simulink model "ModeleSimulinkQ20_2016a"  (R2016a)
settings: Solver=VariableStepAuto  SolverMode=SingleTasking  StartTime=0.0  StopTime=500  RelTol=1e-3
values from neighbouring files (symbols this model uses):
  qdf = [0 1 0 0 0 0]'    [TP2.m]
  qdi = [-1 0 -1 -1 -1 -1]'    [TP2.m]
libraries: simulink x1
settings Model: Creator=davide  LastModifiedBy=davide
settings DataIOCC: ReturnWorkspaceOutputs=on
settings DebuggingCC: SFUnexpectedBacktrackingDiag=error  SFNoUnconditionalDefaultTransitionDiag=error
settings SFSimCC: SimUseLocalCustomCode=on
settings RTWCC: RTWUseLocalCustomCode=on
settings GRTTargetCC: TargetLangStandard=C99 (ISO)  GeneratePreprocessorConditionals=Use local settings
settings ConfigComp: CovMetricSettings=dwe  CovHtmlReporting=off  CovSaveCumulativeToWorkspaceVar=off  CovSaveSingleToWorkspaceVar=off  CovExternalEMLEnable=on

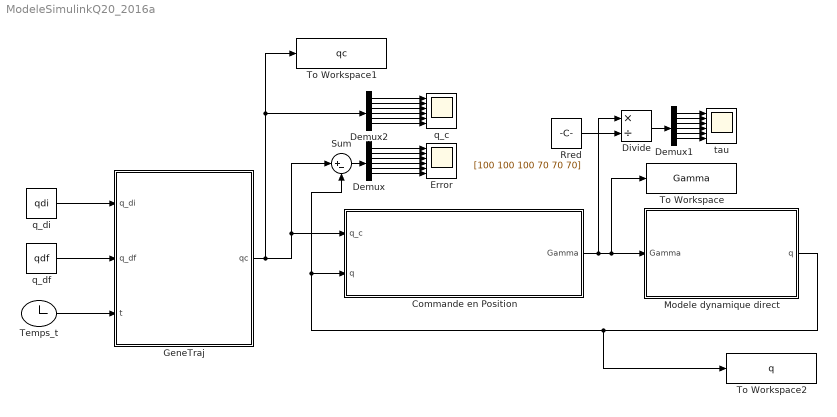
== system ModeleSimulinkQ20_2016a ==
  Commande en Position : Subsystem
  Demux : Demux  Outputs=6
  Demux1 : Demux  Outputs=6
  Demux2 : Demux  Outputs=6
  Divide : Product  Inputs=*/
  Error : Scope  NumInputPorts=6
  GeneTraj : MATLAB Function  TreatAsAtomicUnit=on
  Modele dynamique direct : Subsystem
  Rred : Constant  Value=[100 100 100 70 70 70]
  Sum : Sum  Inputs=|+-
  "Temps_t " : Clock
  To Workspace : ToWorkspace  VariableName=Gamma  SaveFormat=Timeseries  SampleTime=-1
  To Workspace1 : ToWorkspace  VariableName=qc  SaveFormat=Timeseries  SampleTime=-1
  To Workspace2 : ToWorkspace  VariableName=q  SaveFormat=Timeseries  SampleTime=-1
  q_c : Scope  NumInputPorts=6
  "q_df " : Constant  Value=qdf  VectorParams1D=off
  q_di : Constant  Value=qdi  VectorParams1D=off
  tau : Scope  NumInputPorts=6
  wires:
  GeneTraj/1(qc) -> Demux2/1, To Workspace1/1, Sum/1, Commande en Position/1(q_c)
  "Temps_t "/1 -> GeneTraj/3(t)
  "q_df "/1 -> GeneTraj/2(q_df)
  q_di/1 -> GeneTraj/1(q_di)
  Commande en Position/1(Gamma) -> Divide/1, To Workspace/1, Modele dynamique direct/1(Gamma)
  Modele dynamique direct/1(q) -> To Workspace2/1, Sum/2, Commande en Position/2(q)
  Sum/1 -> Demux/1
  Demux/4 -> Error/4
  Demux/1 -> Error/1
  Demux/2 -> Error/2
  Demux/3 -> Error/3
  Demux/5 -> Error/5
  Demux/6 -> Error/6
  Demux2/2 -> q_c/2
  Demux2/6 -> q_c/6
  Demux2/4 -> q_c/4
  Demux2/5 -> q_c/5
  Demux2/3 -> q_c/3
  Demux2/1 -> q_c/1
  Demux1/3 -> tau/3
  Demux1/5 -> tau/5
  Demux1/4 -> tau/4
  Demux1/2 -> tau/2
  Demux1/6 -> tau/6
  Demux1/1 -> tau/1
  Divide/1 -> Demux1/1
  Rred/1 -> Divide/2

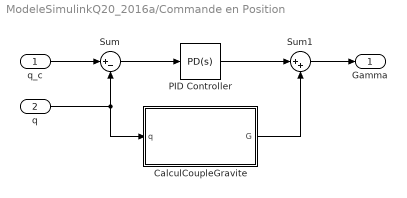
== system ModeleSimulinkQ20_2016a/Commande en Position ==
  q_c : Inport
  q : Inport  Port=2
  CalculCoupleGravite : MATLAB Function  TreatAsAtomicUnit=on
  PID Controller : simulink/Continuous/PID Controller  Controller=PD  Form=Parallel  TimeDomain=Continuous-time  SampleTime=-1  IntegratorMethod=Forward Euler  FilterMethod=Forward Euler  ControllerParametersSource=internal  P=1  I=0  D=0.4  UseFilter=on  N=100  InitialConditionSource=internal  InitialConditionForIntegrator=0  InitialConditionForFilter=0  DifferentiatorICPrevScaledInput=0  ExternalReset=none  TrackingMode=off  Kt=1  LimitOutput=off  UpperSaturationLimit=inf  LowerSaturationLimit=-inf  LinearizeAsGain=on  AntiWindupMode=none  Kb=1  POutMin=[]  POutMax=[]  IOutMin=[]  IOutMax=[]  DOutMin=[]  DOutMax=[]  NOutMin=[]  NOutMax=[]  SumOutMin=[]  SumOutMax=[]  SaturationOutMin=[]  SaturationOutMax=[]  PParamMin=[]  PParamMax=[]  IParamMin=[]  IParamMax=[]  DParamMin=[]  DParamMax=[]  NParamMin=[]  NParamMax=[]  KbParamMin=[]  KbParamMax=[]  KtParamMin=[]  KtParamMax=[]  KbOutMin=[]  KbOutMax=[]  KtOutMin=[]  KtOutMax=[]  IntegratorOutMin=[]  IntegratorOutMax=[]  FilterOutMin=[]  FilterOutMax=[]  SumI1OutMin=[]  SumI1OutMax=[]  SumI2OutMin=[]  SumI2OutMax=[]  SumI3OutMin=[]  SumI3OutMax=[]  SumDOutMin=[]  SumDOutMax=[]  DifferentiatorOutMin=[]  DifferentiatorOutMax=[]  IntegratorContinuousStateAttributes=''  IntegratorStateMustResolveToSignalObject=off  IntegratorRTWStateStorageClass=Auto  FilterContinuousStateAttributes=''  FilterStateMustResolveToSignalObject=off  FilterRTWStateStorageClass=Auto
  Sum : Sum  Inputs=|+-
  Sum1 : Sum  Inputs=|++
  Gamma : Outport
  wires:
  q/1 -> CalculCoupleGravite/1(q), Sum/2
  q_c/1 -> Sum/1
  Sum/1 -> PID Controller/1
  PID Controller/1 -> Sum1/1
  Sum1/1 -> Gamma/1
  CalculCoupleGravite/1(G) -> Sum1/2

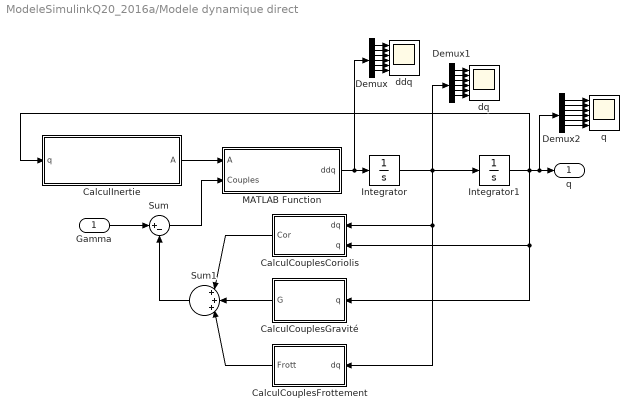
== system ModeleSimulinkQ20_2016a/Modele dynamique direct ==
  Gamma : Inport
  CalculCouplesCoriolis : MATLAB Function  TreatAsAtomicUnit=on
  CalculCouplesFrottement : MATLAB Function  TreatAsAtomicUnit=on
  CalculCouplesGravité : MATLAB Function  TreatAsAtomicUnit=on
  CalculInertie : MATLAB Function  TreatAsAtomicUnit=on
  Demux : Demux  Outputs=6
  Demux1 : Demux  Outputs=6
  Demux2 : Demux  Outputs=6
  Integrator : Integrator
  Integrator1 : Integrator  InitialCondition=[-1 0 -1 -1 -1 -1]'
  MATLAB Function : MATLAB Function  TreatAsAtomicUnit=on
  Sum : Sum  Inputs=|+-
  Sum1 : Sum  Inputs=|+++|
  "ddq " : Scope  NumInputPorts=6
  dq : Scope  NumInputPorts=6
  "q " : Scope  NumInputPorts=6
  q : Outport
  wires:
  Integrator1/1 -> CalculCouplesGravité/1(q), CalculCouplesCoriolis/2(q), CalculInertie/1(q), Demux2/1, q/1
  Integrator/1 -> CalculCouplesFrottement/1(dq), CalculCouplesCoriolis/1(dq), Demux1/1, Integrator1/1
  Gamma/1 -> Sum/1
  CalculInertie/1(A) -> MATLAB Function/1(A)
  Sum/1 -> MATLAB Function/2(Couples)
  MATLAB Function/1(ddq) -> Demux/1, Integrator/1
  Demux/1 -> "ddq "/1
  Demux/2 -> "ddq "/2
  Demux/3 -> "ddq "/3
  Demux/4 -> "ddq "/4
  Demux/5 -> "ddq "/5
  Demux/6 -> "ddq "/6
  Demux1/2 -> dq/2
  Demux1/4 -> dq/4
  Demux1/6 -> dq/6
  Demux1/3 -> dq/3
  Demux1/5 -> dq/5
  Demux1/1 -> dq/1
  Demux2/4 -> "q "/4
  Demux2/1 -> "q "/1
  Demux2/6 -> "q "/6
  Demux2/5 -> "q "/5
  Demux2/2 -> "q "/2
  Demux2/3 -> "q "/3
  Sum1/1 -> Sum/2
  CalculCouplesFrottement/1(Frott) -> Sum1/3
  CalculCouplesGravité/1(G) -> Sum1/2
  CalculCouplesCoriolis/1(Cor) -> Sum1/1

== matlab function ModeleSimulinkQ20_2016a/Commande en Position/CalculCoupleGravite ==
  data: q input; G output
function G = CalculCoupleGravite(q)

    %Parametres
    m=[15 10 1 7 1 0.5];
    x_G1 = 0; y_G1 = 0; z_G1 = -0.25;
    x_G2 = 0.35; y_G2 = 0; z_G2 = 0;
    x_G3 = 0; y_G3 = -0.1; z_G3 = 0;
    x_G4 = 0; y_G4 = 0; z_G4 = 0;
    x_G5 = 0; y_G5 = 0; z_G5 = 0;
    x_G6 = 0; y_G6 = 0; z_G6 = 0;
    x_G = [x_G1 x_G2 x_G3 x_G4 x_G5 x_G6];
    y_G = [y_G1 y_G2 y_G3 y_G4 y_G5 y_G6];
    z_G = [z_G1 z_G2 z_G3 z_G4 z_G5 z_G6];

    d = [0 0 0.7 0 0 0];
    r = [0.5 0 0 0.2 0 0];
    alpha = [0 pi/2 0 pi/2 -pi/2 pi/2];
    theta = [q(1) q(2) q(3)+pi/2 q(4) q(5) q(6)];

    % Calcul des matrices jacobiennes de chacun des corps
    [OJv_Gi, ~] = CalculMatriceJacobienneGi(alpha, d, theta, r, x_G, y_G, z_G);

    %Vecteur gravité exprimé dans R0
    g = [0 0 -9.81]';

    %Calcul du couple de gravité produit par les corps
    G = zeros(length(theta), 1);
    
    for i = 1:length(m)
        G = G - OJv_Gi(:,:,i)'*m(i)*g;
    end
end

== matlab function ModeleSimulinkQ20_2016a/GeneTraj ==
  data: q_di input; qc output; q_df input; t input
function qc = GeneTraj(q_di, q_df, t)
    
    tf = 500;
     
    D = (q_df - q_di);
    
    r = 10 * (t/tf)^3 - 15 * (t/tf)^4 + 6 * (t/tf)^5;
    
    qc = q_di + r*D;
end

== matlab function ModeleSimulinkQ20_2016a/Modele dynamique direct/CalculCouplesCoriolis ==
  data: dq input; q input; Cor output
function Cor = fcn(dq, q)

    Cor = CalculCoupleCoriolisCentrifuge(q, dq)'; 

end

== matlab function ModeleSimulinkQ20_2016a/Modele dynamique direct/CalculInertie ==
  data: q input; A output
function A = CalculMatriceInertie(q)


    %Parametres
    m=[15 10 1 7 1 0.5];
    
    x_G1 = 0; y_G1 = 0; z_G1 = -0.25;
    x_G2 = 0.35; y_G2 = 0; z_G2 = 0;
    x_G3 = 0; y_G3 = -0.1; z_G3 = 0;
    x_G4 = 0; y_G4 = 0; z_G4 = 0;
    x_G5 = 0; y_G5 = 0; z_G5 = 0;
    x_G6 = 0; y_G6 = 0; z_G6 = 0;
    x_G = [x_G1 x_G2 x_G3 x_G4 x_G5 x_G6]';
    y_G = [y_G1 y_G2 y_G3 y_G4 y_G5 y_G6]';
    z_G = [z_G1 z_G2 z_G3 z_G4 z_G5 z_G6]';

    iI = zeros(3,3,6); % pour simulink
    iI(:,:,1)=[0.80 0 0.05 ; 0 0.80 0 ; 0.05  0  0.10];
    iI(:,:,2)=[0.10  0  0.10; 0  1.50 0 ; 0.10  0  1.50];
    iI(:,:,3)=[0.05 0 0 ; 0 0.01 0 ; 0 0 0.05];
    iI(:,:,4)=[0.50 0 0 ; 0 0.50 0 ; 0 0 0.05];
    iI(:,:,5)=[0.01 0 0 ; 0 0.01 0 ; 0 0 0.01];
    iI(:,:,6)=[0.01 0 0 ; 0 0.01 0 ; 0 0 0.01];
    
    d = [0 0 0.7 0 0 0];
    r = [0.5 0 0 0.2 0 0];
    alpha = [0 pi/2 0 pi/2 -pi/2 pi/2];
    theta = [q(1) q(2) q(3)+pi/2 q(4) q(5) q(6)]';
    
    Rred = [100 100 100 70 70 70];
    Jm = 1e-6*[1 1 1 1 1 1];
    %initialisation des tableaux
    g_0i = eye(4);
    Ig = zeros(3*size(q,1),3);
    A = zeros(size(q,1),size(q,1));
    
    %Calcul des matrices jacobiennes de chacun corps
    [OJv_Gi, OJ_wi] = CalculMatriceJacobienneGi(alpha, d, theta, r, x_G, y_G, z_G);
    
    for i = 1 : length(q)
        % Théoreme de Huygens generalisé
        % equation pag 144
        Huygens = [((y_G(i))^2+(z_G(i))^2) -(x_G(i)*y_G(i)) -(x_G(i)*z_G(i));...
                -(x_G(i)*y_G(i)) ((x_G(i))^2+(z_G(i))^2) -(y_G(i)*z_G(i));...
                -(x_G(i)*z_G(i)) -(y_G(i)*z_G(i)) ((x_G(i))^2+(y_G(i))^2);];
    
        %Transport du tenseur d'inertie dans le repère R0
        g_elem = CalculTransformationElem(alpha(i),d(i),theta(i),r(i));
        g_0i = g_0i*g_elem;
        ROi = g_0i(1:3,1:3);
        % Application theoreme de Huygens generalisé
        iI_Gi = iI(:,:,i) + m(i) * Huygens;
        % Retour dans le repere qui nous interesse
        OI_Gi = ROi' * iI_Gi * ROi;
        % Calcul matrice d'inertie du manipulateur
        A = A + ((m(i)*OJv_Gi(:,:,i)')*OJv_Gi(:,:,i) + (OJ_wi(:,:,i)')*OI_Gi*OJ_wi(:,:,i));
    end
    
    %Ajout des contributions des inerties des actionneurs
    A = A + diag(Rred.^2.*Jm);
    
end

== matlab function ModeleSimulinkQ20_2016a/Modele dynamique direct/MATLAB Function ==
  data: A input; ddq output; Couples input
function ddq = fcn(A, Couples)

ddq = inv(A)*Couples;
end

== matlab function ModeleSimulinkQ20_2016a/Modele dynamique direct/CalculCouplesGravité ==
  data: q input; G output
function G = fcn(q)
    
    G = CalculCoupleGravite(q);

end

== matlab function ModeleSimulinkQ20_2016a/Modele dynamique direct/CalculCouplesFrottement ==
  data: dq input; Frott output
function Frott = fcn(dq)

    Frott = CalculCoupleFrottement(dq);
   
end
